simulink model "Power_up_state_machine"  (R2024b)
settings: Solver=FixedStepDiscrete  StartTime=0.0  StopTime=10.0  FixedStep=0.1  RelTol=1e-3  EnableMultiTasking=on
settings Model: Creator=pgoshomi  LastModifiedBy=pgoshomi
settings SolverCC: AlgebraicLoopSolver=TrustRegion  AutoInsertRateTranBlk=on
settings DataIOCC: LimitDataPoints=on
settings OptimizationCC: LifeSpan=inf
settings DebuggingCC: UnconnectedInputMsg=warning  UnconnectedOutputMsg=warning  UnconnectedLineMsg=warning  AllowSymbolicDim=off  SFUnexpectedBacktrackingDiag=warning  SFNoUnconditionalDefaultTransitionDiag=warning  SFExecutionAtInitializationDiag=none  ArithmeticOperatorsInVariantConditions=warning
settings ModelReferenceCC: EnableRefExpFcnMdlSchedulingChecks=on
settings SFSimCC: SimUseLocalCustomCode=off  CustomCodeUndefinedFunction=UseInterfaceOnly
settings RTWCC: RTWUseLocalCustomCode=off  GPUComputeCapability=3.5  DLArmComputeVersion=19.05
settings CodeAppCC: StateflowObjectComments=on
settings GRTTargetCC: TargetLangStandard=C89/C90 (ANSI)
settings ConfigComp: CovMetricSettings=dw  CovSaveCumulativeToWorkspaceVar=on  CovSaveSingleToWorkspaceVar=on  CovExternalEMLEnable=off  CovSFcnEnable=off

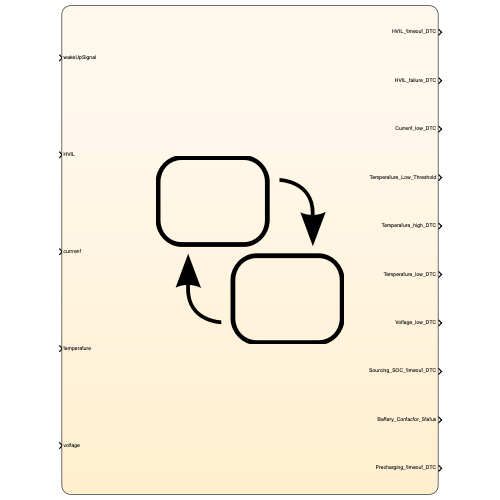
[thumbnail: Simulink's stored preview of the top-level diagram]
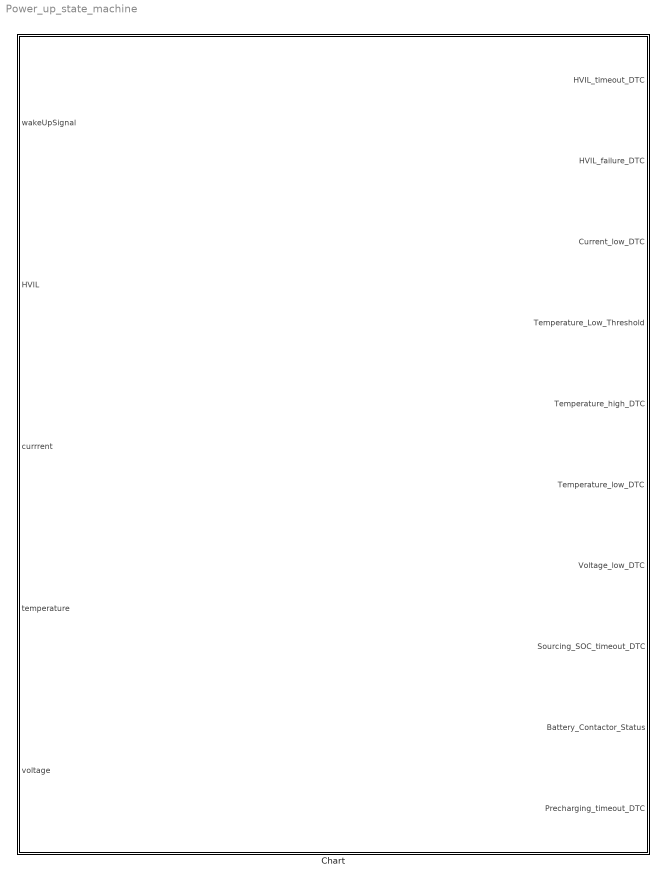
== system Power_up_state_machine ==
  Chart : Stateflow chart  TreatAsAtomicUnit=on

== stateflow chart Power_up_state_machine/Chart ==
  state Sleep
    entry:
    Battery_Contactor_Status = "OPEN"
  state HVIL_source
  state Initialization_Failed
    entry:
    HVIL_failure_DTC = (HVIL == "FAIL");
    HVIL_timeout_DTC = after(60, msec);
    Sourcing_SOC_timeout_DTC = after(160, msec);
    Precharging_timeout_DTC = 1;
  state Source_V_I_SOC
    entry:
    Voltage_low_DTC = voltage <= Voltage_Low_Threshold;
    Current_low_DTC = currrent <= Current_Low_Threshold;
    Temperature_low_DTC = temperature <= Temperature_Low_Threshold;
    Temperature_high_DTC = temperature <= Temperature_High_Threshold;
  state Precharging
  state Contactors_closed
    entry:
    Battery_Contactor_Status = "CLOSE"
  (default) -> Sleep
  Sleep -> HVIL_source : [wakeUpSignal == 12;]
  HVIL_source -> Initialization_Failed [order 2] : [HVIL == "FAIL" || after(60, msec);]
  (junction 32) -> Initialization_Failed
  (junction 30) -> (junction 32) : [ after(200, msec)  ||Voltage_low_DTC == true || Current_low_DTC == true || Temperature_low_DTC == true || Temperature_high_DTC == true;]
  HVIL_source -> Source_V_I_SOC [order 1] : [before(60, msec)  && HVIL == "PASS"; ]
  (junction 42) -> Initialization_Failed
  Source_V_I_SOC -> (junction 30) [order 1]
  Source_V_I_SOC -> Precharging [order 2] : [before(200, msec) == true && (Voltage_low_DTC == false && Current_low_DTC == false && Temperature_low_DTC == false && Temperature_high_DTC == false);]
  Precharging -> (junction 42) [order 2] : [after(400, msec)] { }
  Precharging -> Contactors_closed [order 1] : [PrechargeVoltage >= (0.95 * voltage) && before(400, msec) ]{Quality_Contactor_Command = "CLOSE"}
  data: wakeUpSignal input; HVIL_timeout_DTC output; HVIL_failure_DTC output; HVIL input; Current_Low_Threshold local =0; Current_low_DTC output; Temperature_High_Threshold local =100; Temperature_Low_Threshold output =0; Temperature_high_DTC output; Temperature_low_DTC output; Voltage_Low_Threshold local =0; Voltage_low_DTC output; currrent input; temperature input; voltage input; Sourcing_SOC_timeout_DTC output; Battery_Contactor_Status output; PrechargeVoltage local; Quality_Contactor_Command local; Precharging_timeout_DTC output
